simulink model "two_arm_inductive"  (Simulink 7.3)
settings: Solver=ode45  StartTime=0.0  StopTime=0.2  RelTol=1e-3
libraries: powerlib x11, powerlib_extras x2
settings Model: Creator=DELL  LastModifiedBy=DELL

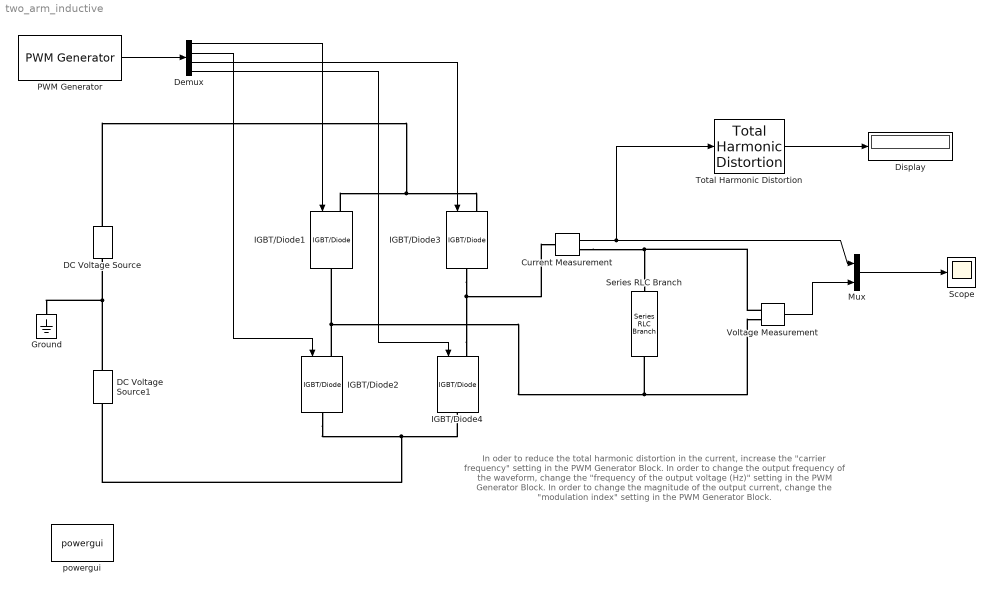
== system two_arm_inductive ==
  note: In oder to reduce the total harmonic distortion in the current, increase the "carrier frequency" setting
      | in the PWM Generator Block.  In order to change the output frequency of the waveform, change the
      | "frequency of the output voltage (Hz)" setting in the PWM Generator Block.  In order to change the
      | magnitude of the output current, change the "modulation index" setting in the PWM Generator Block.
  Current Measurement : powerlib/Measurements/Current Measurement  DialogController=POWERSYS.PowerSysDialog  SystemSampleTime=-1  PhasorSimulation=off  OutputType=Complex  PSBequivalent=0
  DC Voltage Source : powerlib/Electrical Sources/DC Voltage Source  DialogController=POWERSYS.PowerSysDialog  SystemSampleTime=-1  Amplitude=100  Measurements=None
  DC Voltage Source1 : powerlib/Electrical Sources/DC Voltage Source  DialogController=POWERSYS.PowerSysDialog  SystemSampleTime=-1  Amplitude=100  Measurements=None
  Demux : Demux
  Display : Display
  Ground : powerlib/Elements/Ground  DialogController=POWERSYS.PowerSysDialog  PhysicalDomain=powersysdomain  SubClassName=unknown  LeftPortType=p1  RightPortType=p1  LConnTagsString=a
  IGBT/Diode{1..4} (4 alike) : powerlib/Power Electronics/IGBT//Diode  DialogController=POWERSYS.PowerSysDialog  SystemSampleTime=-1  Ron=1e-3  Rs=1e5  Cs=inf  Measurements=off
  Mux : Mux  Inputs=2
  PWM Generator : powerlib_extras/Control  Blocks/PWM Generator  DialogController=POWERSYS.PowerSysDialog  SystemSampleTime=-1  GeneratorMode="2-arm  bridge (4 pulses)"  Fc=1000  Internal=on  mIndex=0.25  Freq=25  Phase=0
  Scope : Scope
  Series RLC Branch : powerlib/Elements/Series RLC Branch  DialogController=POWERSYS.PowerSysDialog  PhysicalDomain=powersysdomain  SubClassName=unknown  LeftPortType=p1  RightPortType=p1  LConnTagsString=__new0  RConnTagsString=__new0  BranchType=RL  Resistance=1  Inductance=5e-3  SetiL0=off  InitialCurrent=0  Capacitance=1e-6  Setx0=off  InitialVoltage=0  Measurements=None
  Total Harmonic Distortion : powerlib_extras/Measurements/Total Harmonic Distortion  DialogController=POWERSYS.PowerSysDialog  SystemSampleTime=-1  f1=50
  Voltage Measurement : powerlib/Measurements/Voltage Measurement  DialogController=POWERSYS.PowerSysDialog  SystemSampleTime=-1  PhasorSimulation=off  OutputType=Complex  PSBequivalent=0
  powergui : powerlib/powergui  Priority=1  SystemSampleTime=-1  SimulationMode=Discrete  SampleTime=5e-6  frequency=60  SPID=off  DisableSnubberDevices=off  DisableRonSwitches=off  DisableVfSwitches=off  SwTol=0  Interpol=off  frequencyindice=0  echomessages=off  HookPort=off  DisplayEquations=off  FunctionMessages=off  EnableUseOfTLC=off  x0status=blocks  RestoreLinks=warning  Frange=[0:2:500]  Ylog=off  Xlog=on  ShowGrid=off  save=off  variable=ZData  ZoomFFT=on  StartTime=0.0  cycles=1  DisplayStyle=1  fundamental=60  FreqAxis=off  MaxFrequency=1000  frequencyindicesteady=1  RmsSteady=1  display=off  Ts=0  methode=off
  wires:
  PWM Generator/1 -> Demux/1
  Mux/1 -> Scope/1
  Voltage Measurement/1 -> Mux/2
  Current Measurement/1 -> Mux/1, Total Harmonic Distortion/1
  Total Harmonic Distortion/1 -> Display/1
  Demux/1 -> IGBT/Diode1/1
  Demux/2 -> IGBT/Diode2/1
  Demux/3 -> IGBT/Diode3/1
  Demux/4 -> IGBT/Diode4/1
  connections:
  IGBT/Diode2/LConn1 -- Series RLC Branch/RConn1 -- Voltage Measurement/LConn2 -- IGBT/Diode1/RConn1
  Voltage Measurement/LConn1 -- Series RLC Branch/LConn1 -- Current Measurement/RConn1
  IGBT/Diode1/LConn1 -- DC Voltage Source/RConn1 -- IGBT/Diode3/LConn1
  IGBT/Diode4/RConn1 -- DC Voltage Source1/LConn1 -- IGBT/Diode2/RConn1
  DC Voltage Source1/RConn1 -- DC Voltage Source/LConn1 -- Ground/LConn1
  IGBT/Diode4/LConn1 -- Current Measurement/LConn1 -- IGBT/Diode3/RConn1
